simulink model "sps_dcdcbuckconverter"  (R2014a)
settings: Solver=ode23tb  StartTime=0.0  StopTime=0.005  FixedStep=1e-08  RelTol=1e-4
PreLoadFcn:
  | Ts = 1e-7;
InitFcn:
  | Ts = 1e-7;
StartFcn:
  | tic;
StopFcn:
  | toc;
libraries: powerlib x11, powerlib_meascontrol x1
settings Model: Creator=cosorio  LastModifiedBy=cosorio
settings DataIOCC: LimitDataPoints=off  SignalLoggingSaveFormat=ModelDataLogs  SaveOutput=off  SignalLogging=off  SaveTime=off
settings OptimizationCC: ExpressionDepthLimit=2147483647
settings DebuggingCC: UnderspecifiedInitializationDetection=Classic  SolverPrmCheckMsg=none  FcnCallInpInsideContextMsg=UseLocalSettings  StateNameClashWarn=warning
settings GRTTargetCC: CombineOutputUpdateFcns=off  GRTInterface=on

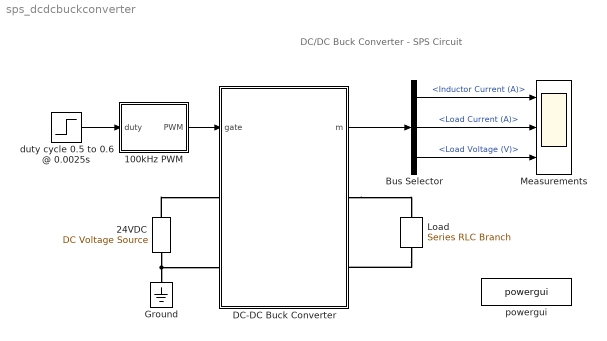
== system sps_dcdcbuckconverter ==
  note: DC/DC Buck Converter - SPS Circuit
  100kHz PWM : Subsystem
  24VDC : powerlib/Electrical Sources/DC Voltage Source  Amplitude=24  Measurements=None
  Bus Selector : BusSelector  OutputSignals=Inductor Current (A),Load Current (A),Load Voltage (V)
  DC-DC Buck Converter : Subsystem
  Ground : powerlib/Elements/Ground  LConnTagsString=a
  Load : powerlib/Elements/Series RLC Branch  LConnTagsString=__new0  RConnTagsString=__new0  BranchType=R  Resistance=2.4  Inductance=30e-6  SetiL0=off  InitialCurrent=0  Capacitance=100e-6  Setx0=off  InitialVoltage=0  Measurements=None
  Measurements : Scope  NumInputPorts=3
      settings: YMin=0~0~0  YMax=10~10~20  SaveName=BuckSPS
  duty cycle 0.5 to 0.6 @ 0.0025s : Step  Time=0.0025  Before=0.5  After=0.6  SampleTime=0
  powergui : powerlib/powergui  Priority=1  SimulationMode=Discrete  SolverType=Tustin  SampleTime=Ts  frequency=60  SPID=off  DisableSnubberDevices=on  DisableRonSwitches=on  DisableVfSwitches=off  SwTol=0  Interpol=off  DisplayEquations=off  Ts=0  methode=off  frequencyindice=0  Pbase=100e6  ErrMax=1e-4  Iterations=50  UnitsV=kV  UnitsW=MW  FunctionMessages=off  echomessages=off  HookPort=off  EnableUseOfTLC=off  x0status=blocks  RestoreLinks=warning  ResistiveCurrentMeasurement=off  Frange=[0:2:500]  Ylog=off  Xlog=on  ShowGrid=off  save=off  variable=ZData  structure=0  ZoomFFT=on  StartTime=0.0  cycles=1  DisplayStyle=1  fundamental=60  FreqAxis=off  MaxFrequency=1000  frequencyindicesteady=1  RmsSteady=1  display=off
  wires:
  DC-DC Buck Converter/1(m) -> Bus Selector/1
  Bus Selector/1 -> Measurements/1  "<Inductor Current (A)>"
  Bus Selector/3 -> Measurements/3  "<Load Voltage (V)>"
  Bus Selector/2 -> Measurements/2  "<Load Current (A)>"
  duty cycle 0.5 to 0.6 @ 0.0025s/1 -> 100kHz PWM/1(duty)
  100kHz PWM/1(PWM) -> DC-DC Buck Converter/1(gate)
  connections:
  24VDC/LConn1 -- Ground/LConn1 -- DC-DC Buck Converter/LConn2
  24VDC/RConn1 -- DC-DC Buck Converter/LConn1
  DC-DC Buck Converter/RConn1 -- Load/RConn1
  Load/LConn1 -- DC-DC Buck Converter/RConn2

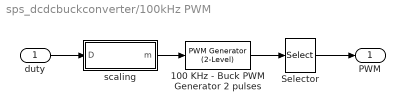
== system sps_dcdcbuckconverter/100kHz PWM ==
  duty : Inport
  100 KHz - Buck PWM Generator 2 pulses : powerlib_meascontrol/Pulse & Signal Generators/PWM Generator (2-Level)  ModulatorType=Single-phase half-bridge (2 pulses)  ModulatorMode=Unsynchronized  nF=27  Fc=1e05  ModulatingSignals=off  m=0.8  Freq=60  Phase=0  Ts=Ts
  Selector : Selector  InputPortWidth=2  Indices=[1]
  scaling : Subsystem
  PWM : Outport
  wires:
  scaling/1(m) -> 100 KHz - Buck PWM Generator 2 pulses/1
  duty/1 -> scaling/1(D)
  100 KHz - Buck PWM Generator 2 pulses/1 -> Selector/1
  Selector/1 -> PWM/1

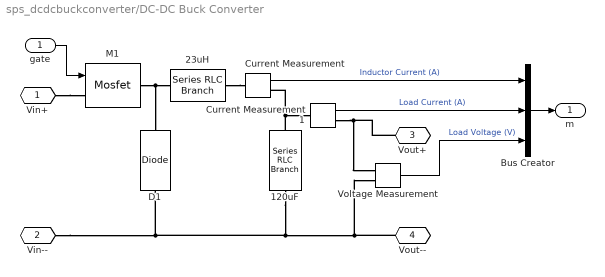
== system sps_dcdcbuckconverter/DC-DC Buck Converter ==
  gate : Inport
  120uF : powerlib/Elements/Series RLC Branch  LConnTagsString=__new0  RConnTagsString=__new0  BranchType=RC  Resistance=0.25  Inductance=30e-6  SetiL0=off  InitialCurrent=0  Capacitance=120e-6  Setx0=off  InitialVoltage=0  Measurements=None
  23uH : powerlib/Elements/Series RLC Branch  LConnTagsString=__new0  RConnTagsString=__new0  BranchType=RL  Resistance=0.05  Inductance=23e-6  SetiL0=off  InitialCurrent=0  Capacitance=1e-6  Setx0=off  InitialVoltage=0  Measurements=None
  Bus Creator : BusCreator  Inputs=3
  Current Measurement : powerlib/Measurements/Current Measurement  PhasorSimulation=off  OutputType=Complex  PSBequivalent=0
  Current Measurement1 : powerlib/Measurements/Current Measurement  PhasorSimulation=off  OutputType=Complex  PSBequivalent=0
  D1 : powerlib/Power Electronics/Diode  Ron=0.01  Lon=0  Vf=0.5  IC=0  UseSnubber=off  Rs=1e5  Cs=250e-9  Measurements=off
  M1 : powerlib/Power Electronics/Mosfet  Ron=0.001  Lon=0  Rd=0.01  Vfd=0.7  IC=0  Rs=1e5  Cs=inf  Measurements=off
  Voltage Measurement : powerlib/Measurements/Voltage Measurement  PhasorSimulation=off  OutputType=Complex  PSBequivalent=0
  Vin+ : PMIOPort  Port=1  Side=Left
  Vin-- : PMIOPort  Port=2  Side=Left
  Vout+ : PMIOPort  Port=3  Side=Right
  Vout-- : PMIOPort  Port=4  Side=Right
  m : Outport
  wires:
  gate/1 -> M1/1
  Current Measurement1/1 -> Bus Creator/2  "Load Current (A)"
  Current Measurement/1 -> Bus Creator/1  "Inductor Current (A)"
  Voltage Measurement/1 -> Bus Creator/3  "Load Voltage (V)"
  Bus Creator/1 -> m/1
  connections:
  M1/RConn1 -- D1/RConn1 -- 23uH/RConn1
  23uH/LConn1 -- Current Measurement/LConn1
  120uF/LConn1 -- Current Measurement1/LConn1 -- Current Measurement/RConn1
  Current Measurement1/RConn1 -- Vout+/RConn1 -- Voltage Measurement/LConn1
  Vin+/RConn1 -- M1/LConn1
  Vin--/RConn1 -- 120uF/RConn1 -- Vout--/RConn1 -- Voltage Measurement/LConn2 -- D1/LConn1

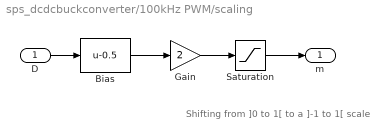
== system sps_dcdcbuckconverter/100kHz PWM/scaling ==
  note: Shifting from ]0 to 1[ to a ]-1 to 1[ scale
  D : Inport
  Bias : Bias  Bias=-0.5
  Gain : Gain  Gain=2
  Saturation : Saturate  UpperLimit=1  LowerLimit=-1
  m : Outport
  wires:
  Bias/1 -> Gain/1
  D/1 -> Bias/1
  Gain/1 -> Saturation/1
  Saturation/1 -> m/1
